simulink model "platform_self_balancing"  (R2024b)
settings: Solver=ode1be  StartTime=0.0  StopTime=10  FixedStep=0.0001  MaxStep=0.0001  RelTol=1e-3
undefined symbols (not defined in the file): fractalcoef, X, Y, Z
libraries: sm_lib x209, nesl_utility x16, slpidlib x1, mspfiltlib x1, mspsensorlib x1
(part 1 of 2)
settings Model: Creator=20844  LastModifiedBy=20844
settings SolverCC: ZeroCrossControl=DisableAll
settings DebuggingCC: AlgebraicLoopMsg=none

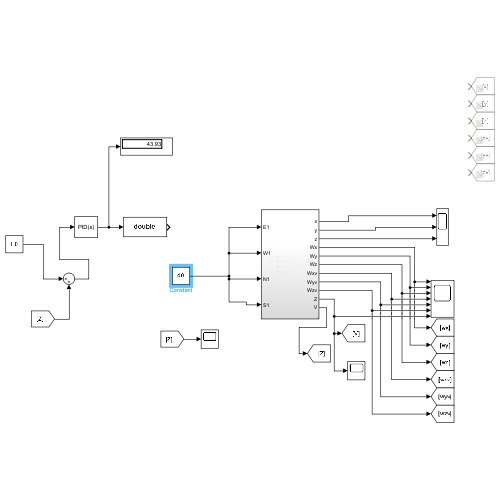
[thumbnail: Simulink's stored preview of the top-level diagram]
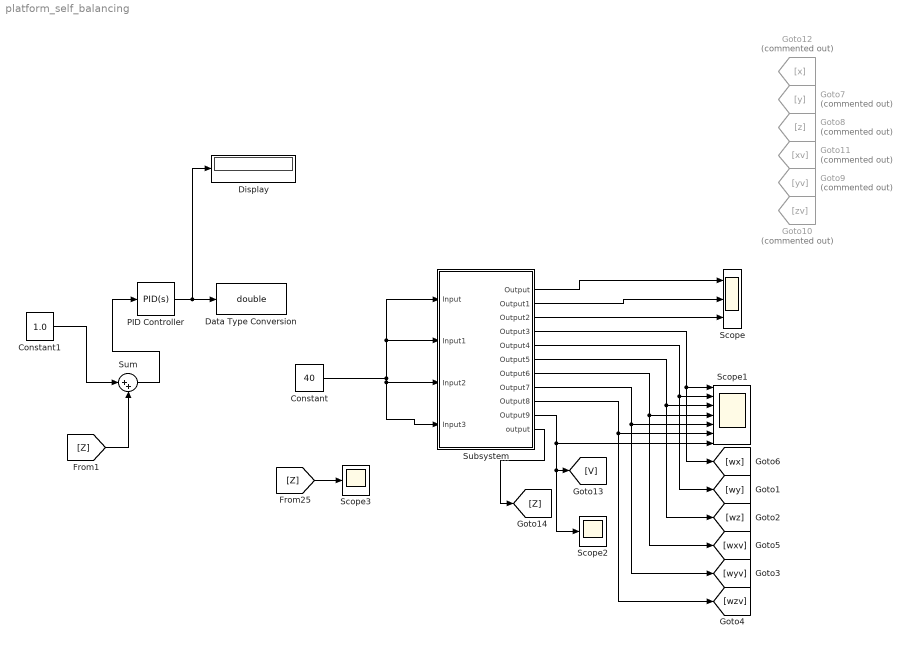
== system platform_self_balancing ==
  Constant : Constant  Value=40
  Constant1 : Constant  Value=1.0
  Data Type Conversion : DataTypeConversion  OutDataTypeStr=double  SaturateOnIntegerOverflow=off  RndMeth=Floor
  Display : Display
  Goto10 : Goto  Commented=on  GotoTag=zv
  Goto11 : Goto  Commented=on  GotoTag=xv
  Goto12 : Goto  Commented=on  GotoTag=x
  Goto7 : Goto  Commented=on  GotoTag=y
  Goto8 : Goto  Commented=on  GotoTag=z
  Goto9 : Goto  Commented=on  GotoTag=yv
  PID Controller : slpidlib/PID Controller  Controller=PID  Form=Parallel  TimeDomain=Continuous-time  UseExternalTs=off  SampleTime=-1  IntegratorMethod=Forward Euler  FilterMethod=Forward Euler  ControllerParametersSource=internal  P=20  I=0  UseKiTs=off  D=0  UseExternalDerivativeSource=off  N=100  UseFilter=on  TunerSelectOption=Transfer Function Based (PID Tuner App)  InitialConditionSource=internal  InitialConditionForIntegrator=0  InitialConditionForFilter=0  DifferentiatorICPrevScaledInput=0  ExternalReset=none  TrackingMode=off  Kt=1  LimitOutput=off  SatLimitsSource=internal  UpperSaturationLimit=inf  LowerSaturationLimit=-inf  LinearizeAsGain=on  AntiWindupMode=none  Kb=1  LimitIntegrator=off  UpperIntegratorSaturationLimit=inf  LowerIntegratorSaturationLimit=-inf  PGainOutDataTypeStr=Inherit: Inherit via back propagation  PProdOutDataTypeStr=Inherit: Inherit via back propagation  POutMin=[]  POutMax=[]  IGainOutDataTypeStr=Inherit: Inherit via back propagation  IProdOutDataTypeStr=Inherit: Inherit via back propagation  IOutMin=[]  IOutMax=[]  DGainOutDataTypeStr=Inherit: Inherit via back propagation  DProdOutDataTypeStr=Inherit: Inherit via back propagation  DOutMin=[]  DOutMax=[]  NGainOutDataTypeStr=Inherit: Inherit via back propagation  NProdOutDataTypeStr=Inherit: Inherit via back propagation  NOutMin=[]  NOutMax=[]  SumOutDataTypeStr=Inherit: Inherit via back propagation  SumOutMin=[]  SumOutMax=[]  SaturationOutMin=[]  SaturationOutMax=[]  PParamMin=[]  PParamMax=[]  IParamMin=[]  IParamMax=[]  DParamMin=[]  DParamMax=[]  NParamMin=[]  NParamMax=[]  KbParamMin=[]  KbParamMax=[]  KtParamMin=[]  KtParamMax=[]  KbOutMin=[]  KbOutMax=[]  KtOutMin=[]  KtOutMax=[]  IntegratorOutMin=[]  IntegratorOutMax=[]  FilterOutMin=[]  FilterOutMax=[]  SumI1OutMin=[]  SumI1OutMax=[]  SumI2OutMin=[]  SumI2OutMax=[]  SumI3OutMin=[]  SumI3OutMax=[]  SumI4OutMin=[]  SumI4OutMax=[]  SumDOutMin=[]  SumDOutMax=[]  DifferentiatorOutMin=[]  DifferentiatorOutMax=[]  FilterDiffOutCoefMin=[]  FilterDiffOutCoefMax=[]  ReciprocalOutMin=[]  ReciprocalOutMax=[]  SumDenOutMin=[]  SumDenOutMax=[]  SumNumOutMin=[]  SumNumOutMax=[]  DivideOutMin=[]  DivideOutMax=[]  UdiffTsProdOutMin=[]  UdiffTsProdOutMax=[]  NTsProdOutMin=[]  NTsProdOutMax=[]  UintegralTsProdOutMin=[]  UintegralTsProdOutMax=[]  UngainTsProdOutMin=[]  UngainTsProdOutMax=[]  ClampingZeroOutDataTypeStr=Inherit: Inherit via back propagation  ClampingZeroOutMin=[]  ClampingZeroOutMax=[]  FilterDenConstantOutDataTypeStr=Inherit: Inherit via back propagation  FilterDenConstantOutMin=[]  FilterDenConstantOutMax=[]  PCopyOutDataTypeStr=Inherit: Inherit via back propagation  PCopyOutMin=[]  PCopyOutMax=[]  NCopyOutDataTypeStr=Inherit: Inherit via back propagation  NCopyOutMin=[]  NCopyOutMax=[]  IntegratorContinuousStateAttributes=''  IntegratorStateMustResolveToSignalObject=off  IntegratorRTWStateStorageClass=Auto  FilterContinuousStateAttributes=''  FilterStateMustResolveToSignalObject=off  FilterRTWStateStorageClass=Auto  ParallelPVariant=InternalParameters  IdealPVariant=Disabled  IVariant=InternalParameters  DVariant=InternalParameters  IntegratorVariant=Continuous  SatVariant=Disabled  AWVariant=Passthrough  PCopyVariant=Disabled  TRVariant=Disabled  FdbkBlocksVariant=Forward  IdealPFdbkVariant=Disabled  SatFdbkVariant=Disabled  DerivativeFilterVariant=ContFilter  NVariant=InternalParameters  NCopyVariant=Disabled  FilterICVariant=InternalICsFilter  IntegratorICVariant=InternalICs  ExternalResetVariant=Disabled  TRSumVariant=Passthrough  SumFdbkVariant=Disabled  SumVariant=Sum_PID  TsampFilterVariant=InternalTs  TsampNgainVariant=Passthrough  TsampIntegralVariant=Disabled_SignalSpec  ExternalSaturationOutDataTypeStr=Inherit: Same as second input  DerivativeSourceVariant=ErrorSignal  PreIntVariant=InternalPreInt
  Scope : Scope  NumInputPorts=3
  Scope1 : Scope  NumInputPorts=7
  Scope2 : Scope
  Scope3 : Scope
  Subsystem : Subsystem
  Sum : Sum  Inputs=|++
  wires:
  Subsystem/1(Output) -> Scope/1
  Subsystem/2(Output1) -> Scope/2
  Subsystem/3(Output2) -> Scope/3
  Subsystem/4(Output3) -> [wx], Scope1/1
  Subsystem/5(Output4) -> [wy], Scope1/2
  Subsystem/6(Output5) -> [wz], Scope1/3
  Subsystem/7(Output6) -> [wxv], Scope1/4
  Subsystem/8(Output7) -> [wyv], Scope1/5
  Subsystem/9(Output8) -> [wzv], Scope1/6
  Subsystem/10(Output9) -> Scope2/1, [V], Scope1/7
  Subsystem/11(output) -> [Z]
  [Z] -> Scope3/1
  [Z] -> Sum/2
  Constant1/1 -> Sum/1
  Sum/1 -> PID Controller/1
  Constant/1 -> Subsystem/1(Input), Subsystem/2(Input1), Subsystem/4(Input3), Subsystem/3(Input2)
  PID Controller/1 -> Display/1, Data Type Conversion/1
